simulink subsystem "StudentTemplate_SNGKHA008_M1_sim"  (R2025b)
settings: Solver=VariableStepAuto  StartTime=0.0  StopTime=10.0  RelTol=1e-3
libraries: simulink x4, eeGeneralControl x4, slpidlib x2
settings Model: Creator=JesseJabezArendse  LastModifiedBy=muner

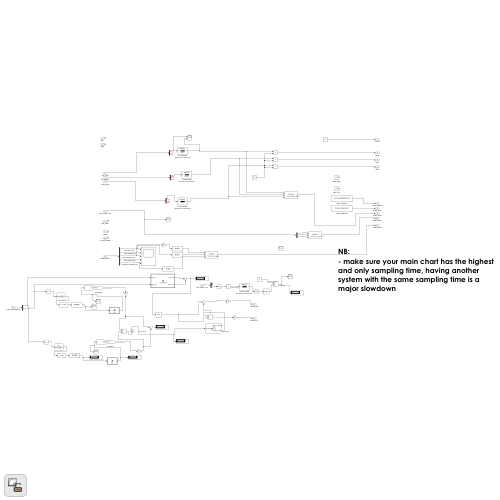
[thumbnail: Simulink's stored preview of the top-level diagram]
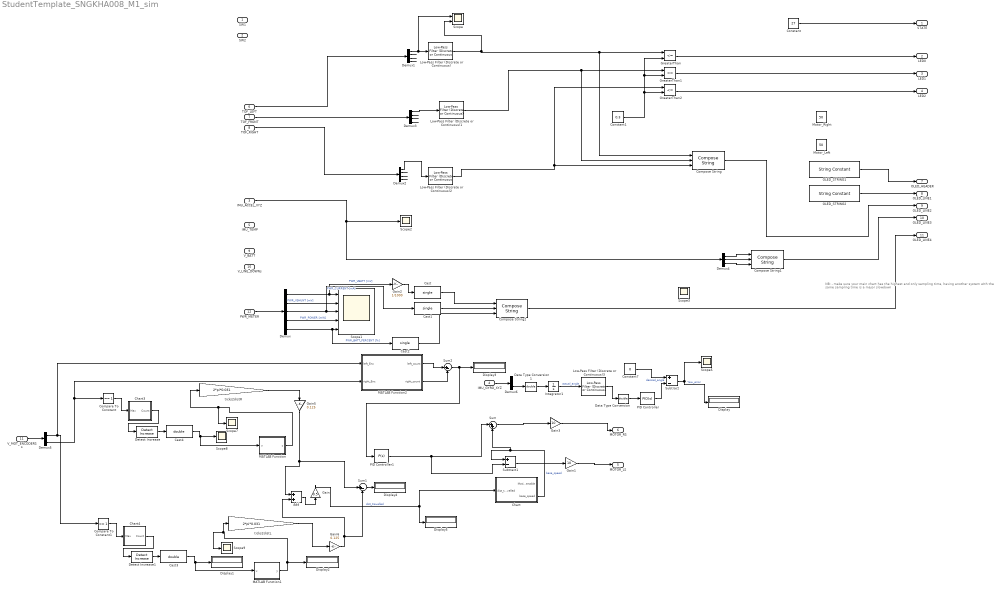
== system StudentTemplate_SNGKHA008_M1_sim ==
  note: NB:
      |
      | - make sure your main chart has the highest and only sampling time, having another system with the same sampling time is a major slowdown
  SW1 : Inport
  SW2 : Inport  Port=2
  IMU_ACCEL_XYZ : Inport  Port=3
  IMU_GYRO_XYZ : Inport  Port=4
  IMU_TEMP : Inport  Port=5
  TOF_LEFT : Inport  Port=6
  TOF_FRONT : Inport  Port=7
  TOF_RIGHT : Inport  Port=8
  V_BATT : Inport  Port=9
  V_LINE_DOWNs : Inport  Port=10
  V_MOT_ENCODERSs : Inport  Port=11
  PWR_METER : Inport  Port=12
  Add : Sum
  Cast : DataTypeConversion  OutDataTypeStr=single  SaturateOnIntegerOverflow=off  RndMeth=Floor
  Cast1 : DataTypeConversion  OutDataTypeStr=single  SaturateOnIntegerOverflow=off  RndMeth=Floor
  Cast2 : DataTypeConversion  OutDataTypeStr=single  SaturateOnIntegerOverflow=off  RndMeth=Floor
  Cast3 : DataTypeConversion  OutDataTypeStr=double  SaturateOnIntegerOverflow=off  RndMeth=Floor
  Cast4 : DataTypeConversion  OutDataTypeStr=double  SaturateOnIntegerOverflow=off  RndMeth=Floor
  Chart : Stateflow chart  TreatAsAtomicUnit=on
  Chart3 : Stateflow chart  TreatAsAtomicUnit=on
  Chart4 : Stateflow chart  TreatAsAtomicUnit=on
  Compare To Constant : simulink/Logic and Bit Operations/Compare To Constant  relop===  const=1  OutDataTypeStr=boolean
  Compare To Constant1 : simulink/Logic and Bit Operations/Compare To Constant  relop===  const=1  OutDataTypeStr=boolean
  Compose String : ComposeString  Format="\"L%1.2f F%1.2f R%1.2f\""
  Compose String1 : ComposeString  Format="\"X%2.1f  Y%2.1f  Z%2.1f\""
  Compose String2 : ComposeString  Format="\"%1.2fV  %3.0fmA  %2.0f%%\""
  Constant : Constant  Value=27
  Constant1 : Constant  Value=0.3  SampleTime=-1
  Constant7 : Constant  Value=0
  Data Type Conversion : DataTypeConversion  OutDataTypeStr=double  SaturateOnIntegerOverflow=off  RndMeth=Floor
  Data Type Conversion1 : DataTypeConversion  OutDataTypeStr=double  SaturateOnIntegerOverflow=off  RndMeth=Floor
  Demux : Demux  Outputs=5
  Demux1 : Demux
  Demux2 : Demux
  Demux3 : Demux
  Demux4 : Demux  Outputs=3
  Demux5 : Demux  Outputs=2
  Demux6 : Demux  Outputs=3
  Detect Increase : simulink/Logic and Bit Operations/Detect Increase  vinit=0.0  OutDataTypeStr=boolean
  Detect Increase1 : simulink/Logic and Bit Operations/Detect Increase  vinit=0.0  OutDataTypeStr=boolean
  Display{,1..5} (6 alike) : Display
  Gain : Gain  Gain=0.5
  Gain1 : Gain  Gain=10
  Gain2 : Gain  Gain=1/1000
  Gain3 : Gain  Gain=10
  Gain5 : Gain  Gain=0.125
  Gain6 : Gain  Gain=0.125
  GreaterThan : RelationalOperator  Operator=<=  OutDataTypeStr=boolean  RndMeth=Simplest  InputSameDT=off
  GreaterThan1 : RelationalOperator  Operator=<=  OutDataTypeStr=boolean  RndMeth=Simplest  InputSameDT=off
  GreaterThan2 : RelationalOperator  Operator=<=  OutDataTypeStr=boolean  RndMeth=Simplest  InputSameDT=off
  Integrator1 : Integrator
  Low-Pass Filter (Discrete or Continuous) : eeGeneralControl/Low-Pass Filter (Discrete or Continuous)  K=1  T=0.1  B=inf  A=-inf  init_option=Inherited from block input  x0=0  Ts=-1
  Low-Pass Filter (Discrete or Continuous)1 : eeGeneralControl/Low-Pass Filter (Discrete or Continuous)  K=1  T=0.1  B=inf  A=-inf  init_option=Inherited from block input  x0=0  Ts=-1
  Low-Pass Filter (Discrete or Continuous)2 : eeGeneralControl/Low-Pass Filter (Discrete or Continuous)  K=1  T=0.1  B=inf  A=-inf  init_option=Inherited from block input  x0=0  Ts=-1
  Low-Pass Filter (Discrete or Continuous)3 : eeGeneralControl/Low-Pass Filter (Discrete or Continuous)  K=2  T=0.1  B=inf  A=-inf  init_option=Inherited from block input  x0=0  Ts=0.01
  MATLAB Function : MATLAB Function  TreatAsAtomicUnit=on
  MATLAB Function1 : MATLAB Function  TreatAsAtomicUnit=on
  MATLAB Function2 : MATLAB Function  TreatAsAtomicUnit=on
  Motor_Left : Constant  Value=50
  Motor_Right : Constant  Value=50
  OLED_STRING1 : StringConstant  String="\"UCT MICROMOUSE '25\""
  OLED_STRING2 : StringConstant  String="\"Simulink Data Demo\""
  PID Controller : slpidlib/PID Controller  Controller=PID  Form=Parallel  TimeDomain=Continuous-time  UseExternalTs=off  SampleTime=-1  IntegratorMethod=Forward Euler  FilterMethod=Forward Euler  ControllerParametersSource=internal  P=1  I=0.1  UseKiTs=off  D=0.01  UseExternalDerivativeSource=off  N=100  UseFilter=on  TunerSelectOption=Frequency Response Based  InitialConditionSource=internal  InitialConditionForIntegrator=0  InitialConditionForFilter=0  DifferentiatorICPrevScaledInput=0  ExternalReset=none  TrackingMode=off  Kt=1  LimitOutput=off  SatLimitsSource=internal  UpperSaturationLimit=inf  LowerSaturationLimit=-inf  LinearizeAsGain=on  AntiWindupMode=none  Kb=1  LimitIntegrator=off  UpperIntegratorSaturationLimit=inf  LowerIntegratorSaturationLimit=-inf  POutMin=[]  POutMax=[]  IOutMin=[]  IOutMax=[]  DOutMin=[]  DOutMax=[]  NOutMin=[]  NOutMax=[]  SumOutMin=[]  SumOutMax=[]  SaturationOutMin=[]  SaturationOutMax=[]  PParamMin=[]  PParamMax=[]  IParamMin=[]  IParamMax=[]  DParamMin=[]  DParamMax=[]  NParamMin=[]  NParamMax=[]  KbParamMin=[]  KbParamMax=[]  KtParamMin=[]  KtParamMax=[]  KbOutMin=[]  KbOutMax=[]  KtOutMin=[]  KtOutMax=[]  IntegratorOutMin=[]  IntegratorOutMax=[]  FilterOutMin=[]  FilterOutMax=[]  SumI1OutMin=[]  SumI1OutMax=[]  SumI2OutMin=[]  SumI2OutMax=[]  SumI3OutMin=[]  SumI3OutMax=[]  SumI4OutMin=[]  SumI4OutMax=[]  SumDOutMin=[]  SumDOutMax=[]  DifferentiatorOutMin=[]  DifferentiatorOutMax=[]  FilterDiffOutCoefMin=[]  FilterDiffOutCoefMax=[]  ReciprocalOutMin=[]  ReciprocalOutMax=[]  SumDenOutMin=[]  SumDenOutMax=[]  SumNumOutMin=[]  SumNumOutMax=[]  DivideOutMin=[]  DivideOutMax=[]  UdiffTsProdOutMin=[]  UdiffTsProdOutMax=[]  NTsProdOutMin=[]  NTsProdOutMax=[]  UintegralTsProdOutMin=[]  UintegralTsProdOutMax=[]  UngainTsProdOutMin=[]  UngainTsProdOutMax=[]  ClampingZeroOutDataTypeStr=Inherit: Inherit via back propagation  ClampingZeroOutMin=[]  ClampingZeroOutMax=[]  FilterDenConstantOutDataTypeStr=Inherit: Inherit via back propagation  FilterDenConstantOutMin=[]  FilterDenConstantOutMax=[]  PCopyOutDataTypeStr=Inherit: Inherit via back propagation  PCopyOutMin=[]  PCopyOutMax=[]  NCopyOutDataTypeStr=Inherit: Inherit via back propagation  NCopyOutMin=[]  NCopyOutMax=[]  IntegratorContinuousStateAttributes=''  IntegratorStateMustResolveToSignalObject=off  IntegratorRTWStateStorageClass=Auto  FilterContinuousStateAttributes=''  FilterStateMustResolveToSignalObject=off  FilterRTWStateStorageClass=Auto  ParallelPVariant=InternalParameters  IdealPVariant=Disabled  IVariant=InternalParameters  DVariant=InternalParameters  IntegratorVariant=Continuous  SatVariant=Disabled  AWVariant=Passthrough  PCopyVariant=Disabled  TRVariant=Disabled  FdbkBlocksVariant=Forward  IdealPFdbkVariant=Disabled  SatFdbkVariant=Disabled  DerivativeFilterVariant=ContFilter  NVariant=InternalParameters  NCopyVariant=Disabled  FilterICVariant=InternalICsFilter  IntegratorICVariant=InternalICs  ExternalResetVariant=Disabled  TRSumVariant=Passthrough  SumFdbkVariant=Disabled  SumVariant=Sum_PID  TsampFilterVariant=InternalTs  TsampNgainVariant=Passthrough  TsampIntegralVariant=Disabled_SignalSpec  ExternalSaturationOutDataTypeStr=Inherit: Same as second input  DerivativeSourceVariant=ErrorSignal  PreIntVariant=InternalPreInt
  PID Controller1 : slpidlib/PID Controller  Controller=P  Form=Parallel  TimeDomain=Continuous-time  UseExternalTs=off  SampleTime=-1  IntegratorMethod=Forward Euler  FilterMethod=Forward Euler  ControllerParametersSource=internal  P=5  I=0.0002  UseKiTs=off  D=0.002  UseExternalDerivativeSource=off  N=100  UseFilter=on  TunerSelectOption=Transfer Function Based (PID Tuner App)  InitialConditionSource=internal  InitialConditionForIntegrator=0  InitialConditionForFilter=0  DifferentiatorICPrevScaledInput=0  ExternalReset=none  TrackingMode=off  Kt=1  LimitOutput=off  SatLimitsSource=internal  UpperSaturationLimit=inf  LowerSaturationLimit=-inf  LinearizeAsGain=on  AntiWindupMode=none  Kb=1  LimitIntegrator=off  UpperIntegratorSaturationLimit=inf  LowerIntegratorSaturationLimit=-inf  POutMin=[]  POutMax=[]  IOutMin=[]  IOutMax=[]  DOutMin=[]  DOutMax=[]  NOutMin=[]  NOutMax=[]  SumOutMin=[]  SumOutMax=[]  SaturationOutMin=[]  SaturationOutMax=[]  PParamMin=[]  PParamMax=[]  IParamMin=[]  IParamMax=[]  DParamMin=[]  DParamMax=[]  NParamMin=[]  NParamMax=[]  KbParamMin=[]  KbParamMax=[]  KtParamMin=[]  KtParamMax=[]  KbOutMin=[]  KbOutMax=[]  KtOutMin=[]  KtOutMax=[]  IntegratorOutMin=[]  IntegratorOutMax=[]  FilterOutMin=[]  FilterOutMax=[]  SumI1OutMin=[]  SumI1OutMax=[]  SumI2OutMin=[]  SumI2OutMax=[]  SumI3OutMin=[]  SumI3OutMax=[]  SumI4OutMin=[]  SumI4OutMax=[]  SumDOutMin=[]  SumDOutMax=[]  DifferentiatorOutMin=[]  DifferentiatorOutMax=[]  FilterDiffOutCoefMin=[]  FilterDiffOutCoefMax=[]  ReciprocalOutMin=[]  ReciprocalOutMax=[]  SumDenOutMin=[]  SumDenOutMax=[]  SumNumOutMin=[]  SumNumOutMax=[]  DivideOutMin=[]  DivideOutMax=[]  UdiffTsProdOutMin=[]  UdiffTsProdOutMax=[]  NTsProdOutMin=[]  NTsProdOutMax=[]  UintegralTsProdOutMin=[]  UintegralTsProdOutMax=[]  UngainTsProdOutMin=[]  UngainTsProdOutMax=[]  ClampingZeroOutDataTypeStr=Inherit: Inherit via back propagation  ClampingZeroOutMin=[]  ClampingZeroOutMax=[]  FilterDenConstantOutDataTypeStr=Inherit: Inherit via back propagation  FilterDenConstantOutMin=[]  FilterDenConstantOutMax=[]  PCopyOutDataTypeStr=Inherit: Inherit via back propagation  PCopyOutMin=[]  PCopyOutMax=[]  NCopyOutDataTypeStr=Inherit: Inherit via back propagation  NCopyOutMin=[]  NCopyOutMax=[]  IntegratorContinuousStateAttributes=''  IntegratorStateMustResolveToSignalObject=off  IntegratorRTWStateStorageClass=Auto  FilterContinuousStateAttributes=''  FilterStateMustResolveToSignalObject=off  FilterRTWStateStorageClass=Auto  ParallelPVariant=InternalParameters  IdealPVariant=Disabled  IVariant=Disabled  DVariant=Disabled  IntegratorVariant=Disabled  SatVariant=Disabled  AWVariant=Disabled  PCopyVariant=Disabled  TRVariant=Disabled  FdbkBlocksVariant=Forward  IdealPFdbkVariant=Disabled  SatFdbkVariant=Disabled  DerivativeFilterVariant=Disabled  NVariant=Disabled  NCopyVariant=Disabled_SignalSpec  FilterICVariant=Disabled  IntegratorICVariant=Disabled  ExternalResetVariant=Disabled  TRSumVariant=Passthrough  SumFdbkVariant=Disabled  SumVariant=Passthrough_P  TsampFilterVariant=InternalTs  TsampNgainVariant=Passthrough  TsampIntegralVariant=Disabled_SignalSpec  ExternalSaturationOutDataTypeStr=Inherit: Same as second input  DerivativeSourceVariant=Disabled  PreIntVariant=InternalPreInt
  Scope : Scope  NumInputPorts=2
      settings: ActiveDisplayYMinimum=0.22759  ActiveDisplayYMaximum=0.52326
  Scope1 : Scope  NumInputPorts=5
      settings: ActiveDisplayYMinimum=-437.5  ActiveDisplayYMaximum=3937.5  DataLoggingVariableName=ScopeData2
  Scope{2..3,5,7..9} (6 alike) : Scope
      Scope3 settings: ActiveDisplayYMinimum=-1  ActiveDisplayYMaximum=1  DataLoggingVariableName=ScopeData4
      Scope5 settings: ActiveDisplayYMinimum=13.8047200158157  ActiveDisplayYMaximum=15.501792864516879  DataLoggingVariableName=ScopeData8
      Scope7 settings: ActiveDisplayYMinimum=34.194505967509976  ActiveDisplayYMaximum=50.493839833256565  DataLoggingVariableName=ScopeData10
      Scope8 settings: ActiveDisplayYMinimum=-1.0332830006305334  ActiveDisplayYMaximum=1.171716999369468  DataLoggingVariableName=ScopeData11
      Scope9 settings: ActiveDisplayYMinimum=31.903676027688604  ActiveDisplayYMaximum=53.746342286267037  DataLoggingVariableName=ScopeData6
  Subtract : Sum  Inputs=+-
  Subtract1 : Sum  Inputs=+-
  Sum : Sum  Inputs=|++
  Sum1 : Sum  Inputs=|+-
  Sum2 : Sum  Inputs=|+-
  ticks2distL : Gain  Gain=2*pi*0.031
  ticks2distR : Gain  Gain=2*pi*0.031
  STATE : Outport
  LED0 : Outport  Port=2
  LED1 : Outport  Port=3
  LED2 : Outport  Port=4
  MOTOR_LS : Outport  Port=5
  MOTOR_RS : Outport  Port=6
  OLED_HEADER : Outport  Port=7
  OLED_LINE1 : Outport  Port=8
  OLED_LINE2 : Outport  Port=9
  OLED_LINE3 : Outport  Port=10
  OLED_LINE4 : Outport  Port=11
  wires:
  TOF_FRONT/1 -> Demux3/1
  OLED_STRING2/1 -> OLED_LINE1/1
  Demux2/1 -> Low-Pass Filter (Discrete or Continuous)2/1
  Demux2/3 -> ?
  Demux2/2 -> ?
  Demux2/4 -> ?
  Compose String1/1 -> OLED_LINE3/1
  Low-Pass Filter (Discrete or Continuous)1/1 -> Compose String/2, GreaterThan1/1
  GreaterThan1/1 -> LED1/1
  Demux3/3 -> ?
  TOF_RIGHT/1 -> Demux2/1
  Demux3/4 -> ?
  Demux3/2 -> ?
  Demux1/2 -> ?
  Demux3/1 -> Low-Pass Filter (Discrete or Continuous)1/1
  OLED_STRING1/1 -> OLED_HEADER/1
  Demux1/1 -> Scope/1, Low-Pass Filter (Discrete or Continuous)/1
  Compose String/1 -> OLED_LINE2/1
  Constant1/1 -> GreaterThan2/2, GreaterThan1/2, GreaterThan/2
  Demux1/4 -> ?
  GreaterThan2/1 -> LED2/1
  TOF_LEFT/1 -> Demux1/1
  GreaterThan/1 -> LED0/1
  Demux1/3 -> ?
  PWR_METER/1 -> Demux/1
  Demux/1 -> Scope1/1, Gain2/1  "PWR_VBATT [mV]"
  Demux/2 -> Scope1/2  "PWR_VSHUNT [mV]"
  Demux/3 -> Scope1/3, Cast1/1  "PWR_CURRENT [mA]"
  Demux/4 -> Scope1/4  "PWR_POWER [mW]"
  Demux/5 -> Scope1/5, Cast2/1  "PWR_BATT_PERCENT [%]"
  IMU_ACCEL_XYZ/1 -> Demux4/1, Scope2/1
  Demux4/1 -> Compose String1/1
  Demux4/2 -> Compose String1/2
  Demux4/3 -> Compose String1/3
  Compose String2/1 -> OLED_LINE4/1
  Gain2/1 -> Cast/1
  Cast/1 -> Compose String2/1
  Cast1/1 -> Compose String2/2
  Cast2/1 -> Compose String2/3
  Low-Pass Filter (Discrete or Continuous)2/1 -> Compose String/3, GreaterThan2/1
  Low-Pass Filter (Discrete or Continuous)/1 -> Scope/2, Compose String/1, GreaterThan/1
  Constant/1 -> STATE/1
  Subtract/1 -> Scope5/1, Display/1  "Yaw_error"
  Data Type Conversion/1 -> PID Controller/1
  Constant7/1 -> Subtract/1  "desired_angle"
  IMU_GYRO_XYZ/1 -> Demux6/1
  Demux6/3 -> Data Type Conversion1/1
  Low-Pass Filter (Discrete or Continuous)3/1 -> Data Type Conversion/1
  Integrator1/1 -> Low-Pass Filter (Discrete or Continuous)3/1  "actual_angle"
  PID Controller/1 -> Subtract/2
  Data Type Conversion1/1 -> Integrator1/1
  Gain/1 -> Chart/1(dist_travelled), Display5/1  "dist_travelled"
  Gain1/1 -> MOTOR_LS/1
  Detect Increase1/1 -> Cast3/1
  Chart4/1(Count) -> Detect Increase1/1
  Gain6/1 -> Add/2, Sum1/2
  Detect Increase/1 -> Cast4/1
  Gain5/1 -> Add/1, Sum1/1
  ticks2distR/1 -> Gain5/1
  Subtract1/1 -> Gain1/1
  Cast3/1 -> Display1/1, MATLAB Function1/1(u)
  MATLAB Function2/2(right_count) -> Sum2/2
  Compare To Constant/1 -> Chart3/1(Max)
  MATLAB Function/1(y) -> ticks2distR/1, Scope7/1
  Sum2/1 -> PID Controller1/1, Display3/1
  Gain3/1 -> MOTOR_RS/1
  Demux5/2 -> Compare To Constant/1, MATLAB Function2/2(right_Enc)
  V_MOT_ENCODERSs/1 -> Demux5/1
  ticks2distL/1 -> Gain6/1
  Demux5/1 -> Compare To Constant1/1, MATLAB Function2/1(left_Enc)
  PID Controller1/1 -> Sum/1, Subtract1/2
  Chart3/1(Count) -> Detect Increase/1
  Chart/2(base_speed) -> Sum/2, Subtract1/1  "base_speed"
  Sum1/1 -> Display4/1
  MATLAB Function2/1(left_count) -> Sum2/1
  Compare To Constant1/1 -> Chart4/1(Max)
  MATLAB Function1/1(y) -> ticks2distL/1, Scope9/1, Display2/1
  Sum/1 -> Gain3/1
  Cast4/1 -> Scope8/1, MATLAB Function/1(u)
  Add/1 -> Gain/1

== matlab function StudentTemplate_SNGKHA008_M1_sim/MATLAB Function2 ==
  settings: updateMethod=DISCRETE
  data: left_count output; left_Enc input; right_count output; right_Enc input
function [left_count, right_count] = countTicks(left_Enc, right_Enc)

persistent prev_left prev_right count_left count_right

% Initialize on first run
if isempty(prev_left)
    prev_left = 0;
    prev_right = 0;
    count_left = 0;
    count_right = 0;
end

%Detect rising edges (0 -> 1)
if (left_Enc == 1) && (prev_left == 0)
    count_left = count_left + 1;
end

if (right_Enc == 1) && (prev_right == 0)
    count_right = count_right + 1;
end

%Update previous signal states
prev_left = left_Enc;
prev_right = right_Enc;

%Output cumulative counts
left_count = count_left;
right_count = count_right;
end

== stateflow chart StudentTemplate_SNGKHA008_M1_sim/Chart ==
  state MoveForward
    entry:
    Motion_enable = true;
    base_speed = 5;
  state Stop
    entry:
    Motion_enable = false;
    base_speed=0;
  (default) -> MoveForward
  MoveForward -> Stop : [dist_travelled>=2]
  data: dist_travelled input; Motion_enable output; base_speed output

== stateflow chart StudentTemplate_SNGKHA008_M1_sim/Chart3 ==
  state Start
    entry:
    Count = 0;
  state Increase
    entry:
    Count = 1;
  (default) -> Start
  Increase -> Start : after(0.2, sec)
  Start -> Increase : [Max==1]
  data: Max input; Count output

== matlab function StudentTemplate_SNGKHA008_M1_sim/MATLAB Function ==
  data: u input; y output

function y = fcn(u)
persistent lastState pulseCounter

% Initialize on first run
if isempty(lastState)
    lastState = false;
    pulseCounter = 0;
end

% Take first element of input
inputVal = u(1);

% Detection threshold
level = 0.5;
aboveLevel = inputVal > level;

% Count only rising transitions
if aboveLevel && ~lastState
    pulseCounter = pulseCounter + 1;
end

% Output current count
y = pulseCounter;

% Update state memory
lastState = aboveLevel;
end

== stateflow chart StudentTemplate_SNGKHA008_M1_sim/Chart4 ==
  state Start
    entry:
    Count = 0;
  state Increase
    entry:
    Count = 1;
  (default) -> Start
  Increase -> Start : after(0.2, sec)
  Start -> Increase : [Max==1]
  data: Max input; Count output

== matlab function StudentTemplate_SNGKHA008_M1_sim/MATLAB Function1 ==
  data: u input; y output
function y = fcn(u)
persistent lastState pulseCounter

% Initialize on first run
if isempty(lastState)
    lastState = false;
    pulseCounter = 0;
end

% Take first element of input
inputVal = u(1);

% Detection threshold
level = 0.5;
aboveLevel = inputVal > level;

% Count only rising transitions
if aboveLevel && ~lastState
    pulseCounter = pulseCounter + 1;
end

% Output current count
y = pulseCounter;

% Update state memory
lastState = aboveLevel;
end
